simulink model "new_fault"  (R2024b)
settings: Solver=VariableStepAuto  StartTime=0.0  StopTime=10.0  RelTol=1e-3
libraries: spsDCVoltageSourceLib x3, spsIGBTDiodeLib x3, spsPWMGeneratorDCDCLib x3, spsCurrentMeasurementLib x1, spsGroundLib x1, spsSeriesRLCBranchLib x1, sps_lib x1
settings Model: Creator=Ranbir  LastModifiedBy=Ranbir

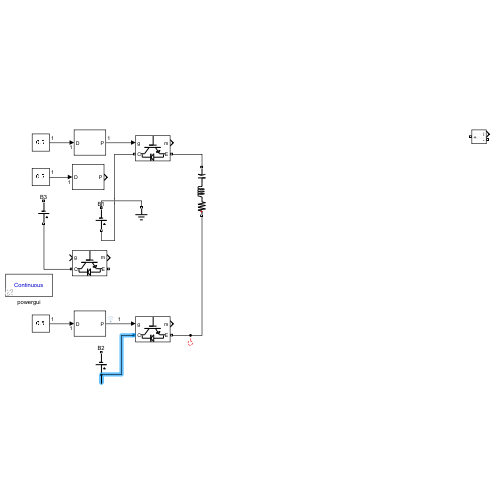
[thumbnail: Simulink's stored preview of the top-level diagram]
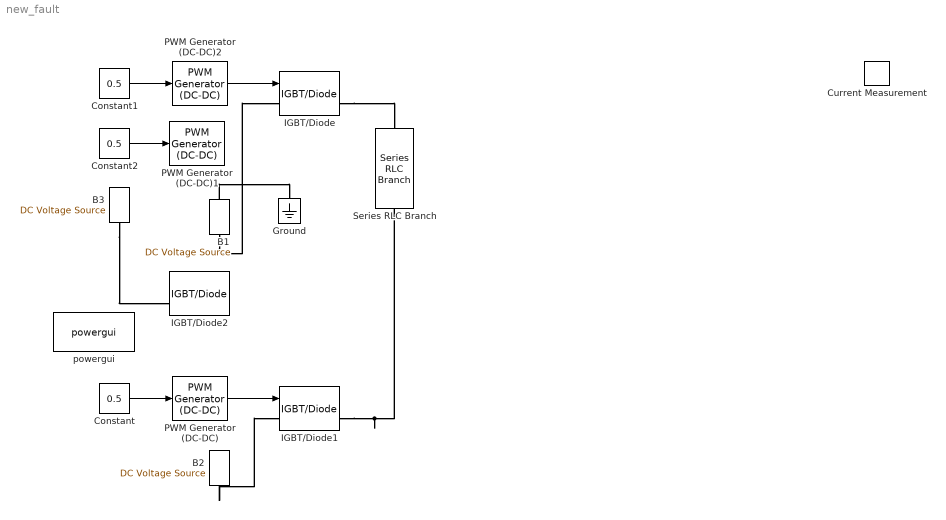
== system new_fault ==
  B1 : spsDCVoltageSourceLib/DC Voltage Source  Amplitude=100  Measurements=None
  B2 : spsDCVoltageSourceLib/DC Voltage Source  Amplitude=100  Measurements=None
  B3 : spsDCVoltageSourceLib/DC Voltage Source  Amplitude=100  Measurements=None
  Constant : Constant  Value=0.5
  Constant1 : Constant  Value=0.5
  Constant2 : Constant  Value=0.5
  Current Measurement : spsCurrentMeasurementLib/Current Measurement  PhasorSimulation=off  OutputType=Complex  PSBequivalent=0
  Ground : spsGroundLib/Ground  LConnTagsString=a
  IGBT/Diode : spsIGBTDiodeLib/IGBT//Diode  Ron=1e-3  Rs=1e5  Cs=inf  Measurements=on
  IGBT/Diode1 : spsIGBTDiodeLib/IGBT//Diode  Ron=1e-3  Rs=1e5  Cs=inf  Measurements=on
  IGBT/Diode2 : spsIGBTDiodeLib/IGBT//Diode  Ron=1e-3  Rs=1e5  Cs=inf  Measurements=on
  PWM Generator (DC-DC) : spsPWMGeneratorDCDCLib/PWM Generator (DC-DC)  Fsw=5000  Ts=1e-6
  PWM Generator (DC-DC)1 : spsPWMGeneratorDCDCLib/PWM Generator (DC-DC)  Fsw=5000  Ts=0
  PWM Generator (DC-DC)2 : spsPWMGeneratorDCDCLib/PWM Generator (DC-DC)  Fsw=5000  Ts=1e-6
  Series RLC Branch : spsSeriesRLCBranchLib/Series RLC Branch  LConnTagsString=__new0  RConnTagsString=__new0  BranchType=RLC  Resistance=10  Inductance=0  SetiL0=off  InitialCurrent=0  Capacitance=0  Setx0=off  InitialVoltage=0  Measurements=None
  powergui : sps_lib/powergui  Priority=1  SimulationMode=Continuous  SampleTime=50e-6  frequency=60  Iterations=50  frequencyindice=0  Pbase=100e6  ErrMax=1e-4  UnitsV=kV  UnitsW=MW  buscounter=0  FunctionMessages=off  echomessages=off  EnableUseOfTLC=off  CurrentSourceSwitches=off  DisableSnubberDevices=off  DisableRonSwitches=off  DisableVfSwitches=off  DisplayEquations=off  AutomaticDiscreteSolvers=off  SolverType=Tustin/Backward Euler (TBE)  Interpol=off  ExternalGateDelay=off  methode=off  Ts=100  x0status=blocks  SPID=on  SwTol=0  HookPort=off  NonlinearTolerance=1e-4  nMaxIteration=100  ContinueOnMaxIteration=off  RestoreLinks=warning  ResistiveCurrentMeasurement=off  Frange=[0:2:500]  Ylog=off  Xlog=on  ShowGrid=off  save=off  variable=ZData  structure=0  ZoomFFT=off  StartTime=0.0  cycles=1  DisplayStyle=1  fundamental=60  FreqAxis=off  MaxFrequency=1000  frequencyindicesteady=1  RmsSteady=1  display=off
  wires:
  Constant/1 -> PWM Generator (DC-DC)/1
  PWM Generator (DC-DC)2/1 -> IGBT/Diode/1
  Constant1/1 -> PWM Generator (DC-DC)2/1
  Constant2/1 -> PWM Generator (DC-DC)1/1
  PWM Generator (DC-DC)/1 -> IGBT/Diode1/1
  connections:
  B1/RConn1 -- IGBT/Diode/LConn1
  B3/RConn1 -- IGBT/Diode2/LConn1
  B2/RConn1 -- IGBT/Diode1/LConn1
  B1/LConn1 -- Ground/LConn1
  IGBT/Diode/RConn1 -- Series RLC Branch/RConn1
  IGBT/Diode1/RConn1 -- Series RLC Branch/LConn1
